simulink model "adaptive_joint_space"  (R2023a)
settings: Solver=VariableStepAuto  StartTime=0.0  StopTime=10.0  RelTol=1e-3
undefined symbols (not defined in the file): A, F, G, I, KD, Ktheta, lambda
settings Model: Creator=franc  LastModifiedBy=franc

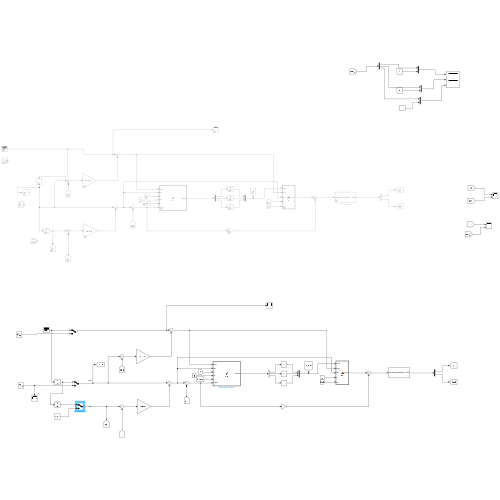
[thumbnail: Simulink's stored preview of the top-level diagram]
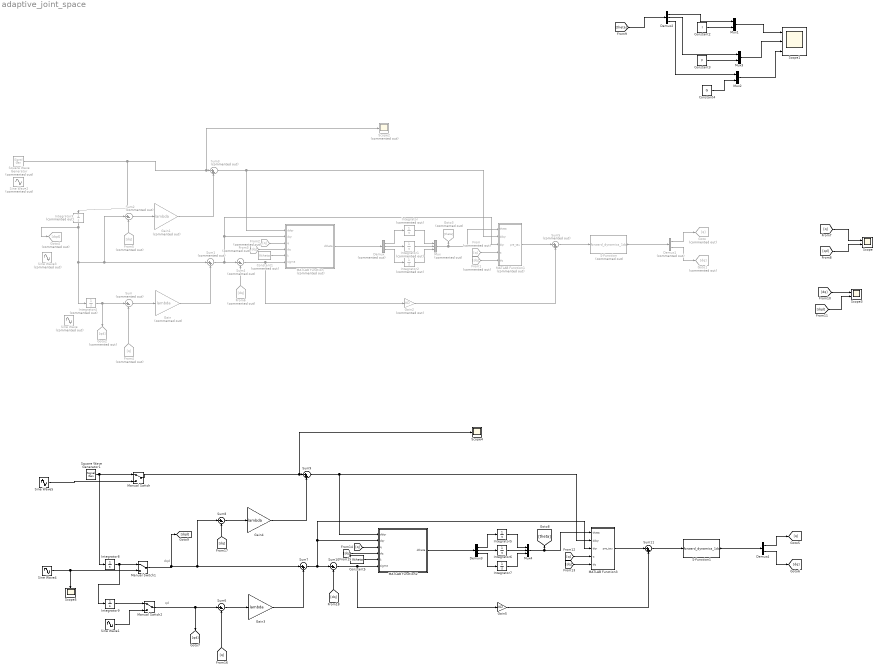
== system adaptive_joint_space ==
  note: qd
  note: dqd
  Constant1 : Constant  Commented=on  Value=Ktheta
  Constant2 : Constant  Value=I
  Constant3 : Constant  Value=F
  Constant4 : Constant  Value=G
  Constant5 : Constant  Value=Ktheta
  Demux : Demux  Commented=on  Outputs=3
  Demux1 : Demux  Commented=on  Outputs=2
  Demux2 : Demux  Outputs=3
  Demux3 : Demux  Outputs=3
  Demux4 : Demux  Outputs=2
  From : From  Commented=on  GotoTag=q
  From{1,3,5..6} (4 alike) : From  Commented=on  GotoTag=dq
  From2 : From  Commented=on  GotoTag=q
  From4 : From  Commented=on  GotoTag=q
  Gain : Gain  Commented=on  Gain=lambda
  Gain1 : Gain  Commented=on  Gain=lambda
  Gain2 : Gain  Commented=on  Gain=KD
  Gain3 : Gain  Gain=lambda
  Gain4 : Gain  Gain=lambda
  Gain5 : Gain  Gain=KD
  Goto : Goto  Commented=on  GotoTag=q
  Goto1 : Goto  Commented=on  GotoTag=dq
  Goto2 : Goto  Commented=on  GotoTag=qd
  Goto3 : Goto  Commented=on  GotoTag=theta
  Goto4 : Goto  Commented=on  GotoTag=dqd
  Integrator : Integrator  Commented=on  InitialCondition=I/2
  Integrator1 : Integrator  Commented=on  InitialCondition=F/2
  Integrator2 : Integrator  Commented=on  InitialCondition=G/2
  Integrator3 : Integrator  Commented=on
  Integrator4 : Integrator  Commented=on
  Integrator5 : Integrator  InitialCondition=I/2
  Integrator6 : Integrator  InitialCondition=F/2
  Integrator7 : Integrator  InitialCondition=G/2
  Integrator8 : Integrator
  Integrator9 : Integrator
  MATLAB Function : MATLAB Function  Commented=on  TreatAsAtomicUnit=on
  MATLAB Function1 : MATLAB Function  Commented=on  TreatAsAtomicUnit=on
  MATLAB Function2 : MATLAB Function  TreatAsAtomicUnit=on
  MATLAB Function3 : MATLAB Function  TreatAsAtomicUnit=on
  Manual Switch : ManualSwitch
  Manual Switch1 : ManualSwitch
  Manual Switch2 : ManualSwitch
  Mux : Mux  Commented=on  Inputs=3
  Mux1 : Mux  Inputs=2
  Mux2 : Mux  Inputs=2
  Mux3 : Mux  Inputs=2
  Mux4 : Mux  Inputs=3
  S-Function : S-Function  Commented=on  FunctionName=forward_dynamics_1dof  Parameters=qi, dqi,I,F,G  SFunctionDeploymentMode=off  EnableBusSupport=off
  S-Function1 : S-Function  FunctionName=forward_dynamics_1dof  Parameters=qi, dqi,I,F,G  SFunctionDeploymentMode=off  EnableBusSupport=off
  Scope : Scope  NumInputPorts=2
  Scope1 : Scope  NumInputPorts=3
  Scope2 : Scope  Commented=on
  Scope3 : Scope  NumInputPorts=2
  Scope4 : Scope
  Scope5 : Scope
  Sine Wave : Sin  Commented=on  Amplitude=A  Frequency=3.14  SampleTime=0
  Sine Wave1 : Sin  Amplitude=A  Frequency=3.14  SampleTime=0
  Sine Wave2 : Sin  Commented=on  Amplitude=-A*3.14*3.14  Frequency=3.14  SampleTime=0
  Sine Wave3 : Sin  Commented=on  Amplitude=A*3.14  Frequency=3.14  Phase=pi/2  SampleTime=0
  Sine Wave4 : Sin  Amplitude=A*3.14  Frequency=3.14  Phase=pi/2  SampleTime=0
  Sine Wave5 : Sin  Amplitude=-A*3.14*3.14  Frequency=3.14  SampleTime=0
  Square Wave Generator : SignalGenerator  Commented=on  WaveForm=square  Amplitude=A  Frequency=2  Units=rad/sec
  Square Wave Generator1 : SignalGenerator  WaveForm=square  Amplitude=A  Frequency=2  Units=rad/sec
  Sum : Sum  Commented=on  Inputs=|+-
  Sum1 : Sum  Commented=on  Inputs=|++
  Sum10 : Sum  Inputs=|+-
  Sum11 : Sum  Inputs=|++
  Sum2 : Sum  Commented=on  Inputs=|+-
  Sum3 : Sum  Commented=on  Inputs=|++
  Sum4 : Sum  Commented=on  Inputs=|+-
  Sum5 : Sum  Commented=on  Inputs=|++
  Sum6 : Sum  Inputs=|+-
  Sum7 : Sum  Inputs=|++
  Sum8 : Sum  Inputs=|+-
  Sum9 : Sum  Inputs=|++
  wires:
  Sum/1 -> Gain/1
  Gain/1 -> Sum1/2
  Integrator3/1 -> Integrator4/1, Sum2/1, Sum1/1, Goto4/1
  Sum2/1 -> Gain1/1
  Gain1/1 -> Sum3/2
  Sum1/1 -> Sum4/1, MATLAB Function1/3(dqr), MATLAB Function/2(dqr)
  Sum4/1 -> MATLAB Function/6(sigma), Gain2/1
  Constant1/1 -> MATLAB Function/5(k)
  Sum3/1 -> MATLAB Function/1(ddqr), MATLAB Function1/2(ddqr)
  MATLAB Function/1(dtheta) -> Demux/1
  Integrator1/1 -> Mux/2
  Demux/2 -> Integrator1/1
  Demux/1 -> Integrator/1
  Demux/3 -> Integrator2/1
  Integrator/1 -> Mux/1
  Integrator2/1 -> Mux/3
  Mux/1 -> Goto3/1, MATLAB Function1/1(theta)
  MATLAB Function1/1(pre_tau) -> Sum5/1
  Sum5/1 -> S-Function/1
  S-Function/1 -> Demux1/1
  Demux1/1 -> Goto/1
  Demux1/2 -> Goto1/1
  From1/1 -> MATLAB Function1/5(dq)
  From/1 -> MATLAB Function1/4(q)
  From2/1 -> MATLAB Function/3(q)
  From3/1 -> MATLAB Function/4(dq)
  From4/1 -> Sum/2
  Gain2/1 -> Sum5/2
  From6/1 -> Sum4/2
  From5/1 -> Sum2/2
  [q] -> Scope/1
  [qd] -> Scope/2
  [theta] -> Demux2/1
  Mux1/1 -> Scope1/1
  Constant2/1 -> Mux1/2
  Demux2/1 -> Mux1/1
  Demux2/2 -> Mux3/1
  Demux2/3 -> Mux2/1
  Constant3/1 -> Mux3/2
  Constant4/1 -> Mux2/2
  Mux2/1 -> Scope1/3
  Mux3/1 -> Scope1/2
  Square Wave Generator/1 -> Scope2/1, Sum3/1, Integrator3/1
  Integrator4/1 -> Goto2/1, Sum/1
  [dq] -> Scope3/1
  [dqd] -> Scope3/2
  Square Wave Generator1/1 -> Manual Switch/1, Integrator8/1
  [dq] -> MATLAB Function2/4(dq)
  Demux3/3 -> Integrator7/1
  Demux4/1 -> [q]
  [dq] -> Sum8/2
  Demux4/2 -> [dq]
  Sum6/1 -> Gain3/1
  Integrator5/1 -> Mux4/1
  Gain3/1 -> Sum7/2
  Sum7/1 -> Sum10/1, MATLAB Function3/3(dqr), MATLAB Function2/2(dqr)
  Sum9/1 -> MATLAB Function2/1(ddqr), MATLAB Function3/2(ddqr)
  Manual Switch1/1 -> [dqd], Sum8/1, Sum7/1
  Integrator7/1 -> Mux4/3
  Manual Switch2/1 -> [qd], Sum6/1
  Constant5/1 -> MATLAB Function2/5(k)
  Gain5/1 -> Sum11/2
  Gain4/1 -> Sum9/2
  Sum11/1 -> S-Function1/1
  Sum8/1 -> Gain4/1
  MATLAB Function2/1(dtheta) -> Demux3/1
  Sum10/1 -> MATLAB Function2/6(sigma), Gain5/1
  Demux3/1 -> Integrator5/1
  MATLAB Function3/1(pre_tau) -> Sum11/1
  Demux3/2 -> Integrator6/1
  [dq] -> Sum10/2
  [dq] -> MATLAB Function3/5(dq)
  [q] -> MATLAB Function2/3(q)
  Integrator6/1 -> Mux4/2
  S-Function1/1 -> Demux4/1
  Mux4/1 -> [theta], MATLAB Function3/1(theta)
  [q] -> MATLAB Function3/4(q)
  [q] -> Sum6/2
  Manual Switch/1 -> Scope4/1, Sum9/1
  Integrator8/1 -> Integrator9/1, Manual Switch1/1
  Integrator9/1 -> Manual Switch2/1
  Sine Wave1/1 -> Manual Switch2/2
  Sine Wave4/1 -> Scope5/1, Manual Switch1/2
  Sine Wave5/1 -> Manual Switch/2

== matlab function adaptive_joint_space/MATLAB Function1 ==
  data: theta input; pre_tau output; ddqr input; dqr input; q input; dq input
function pre_tau = fcn(theta,ddqr,dqr,q,dq)

pre_tau = [ddqr dqr sin(q)] * theta; %slide sx

== matlab function adaptive_joint_space/MATLAB Function ==
  data: ddqr input; dtheta output; dqr input; q input; dq input; k input; sigma input
function dtheta = fcn(ddqr,dqr,q,dq,k,sigma)

dtheta = k*[ddqr;dqr;sin(q)]*(dqr - dq); %slide on the right

== matlab function adaptive_joint_space/MATLAB Function2 ==
  data: ddqr input; dtheta output; dqr input; q input; dq input; k input; sigma input
function dtheta = fcn(ddqr,dqr,q,dq,k,sigma)

dtheta = k*[ddqr;dqr;sin(q)]*(dqr - dq); %slide on the right

== matlab function adaptive_joint_space/MATLAB Function3 ==
  data: theta input; pre_tau output; ddqr input; dqr input; q input; dq input
function pre_tau = fcn(theta,ddqr,dqr,q,dq)

pre_tau = [ddqr dqr sin(q)] * theta; %slide sx
